simulink model "ugvmodel4point"  (R2025b)
settings: Solver=ode45  StartTime=0.0  StopTime=85  RelTol=1e-3
InitFcn:
  | UGVparameters
StopFcn:
  | myAnimation(xActEst,yActEst,thetaAct,X_array,Y_array,rp1,rp2)
  | myPlot(xActEst,yActEst,X_array,Y_array,rp1,rp2)
values from neighbouring files (symbols this model uses):
  b = 0.5842    [UGVparameters.m]
  rL = 0.052959    [UGVparameters.m]
  rR = 0.052959    [UGVparameters.m]
  wmax = Vmax/rR    (= 8.30831397874)    [UGVparameters.m]
settings Model: Creator=vigal  LastModifiedBy=brand
settings SolverCC: AlgebraicLoopSolver=TrustRegion
settings DataIOCC: ReturnWorkspaceOutputs=off
settings DebuggingCC: UnconnectedInputMsg=warning  UnconnectedOutputMsg=warning  UnconnectedLineMsg=warning  ArithmeticOperatorsInVariantConditions=warning
settings ModelReferenceCC: EnableRefExpFcnMdlSchedulingChecks=on
settings SFSimCC: SimUseLocalCustomCode=off  CustomCodeUndefinedFunction=UseInterfaceOnly
settings RTWCC: RTWUseLocalCustomCode=off  GPUComputeCapability=3.5

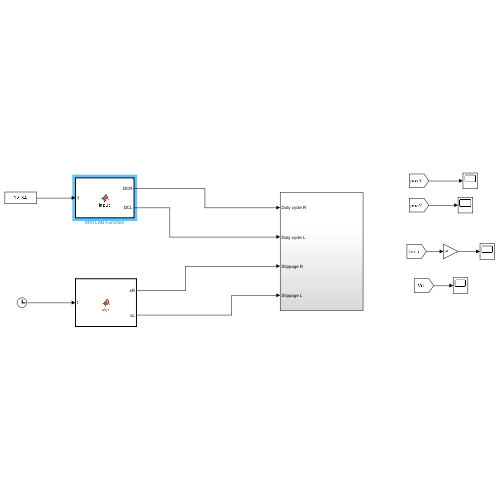
[thumbnail: Simulink's stored preview of the top-level diagram]
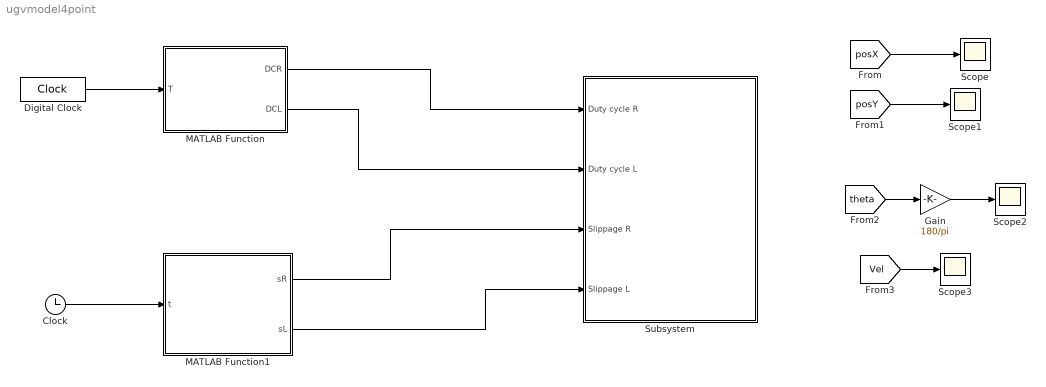
== system ugvmodel4point ==
  Clock : Clock
  Digital Clock : DigitalClock
  Gain : Gain  Gain=180/pi
  MATLAB Function : MATLAB Function  TreatAsAtomicUnit=on
  MATLAB Function1 : MATLAB Function  TreatAsAtomicUnit=on
  Scope{,1..3} (4 alike) : Scope
      Scope settings: ActiveDisplayYMinimum=-0.31428564567099693  ActiveDisplayYMaximum=2.8285708110389729  DataLoggingVariableName=xActEst
      Scope1 settings: ActiveDisplayYMinimum=-1.4039599693481954  ActiveDisplayYMaximum=1.2603387496671137  DataLoggingVariableName=yActEst
      Scope2 settings: ActiveDisplayYMinimum=-1.53363  ActiveDisplayYMaximum=13.80268  DataLoggingVariableName=thetaAct
      Scope3 settings: ActiveDisplayYMinimum=-0.055  ActiveDisplayYMaximum=0.49499  DataLoggingVariableName=ScopeData3
  Subsystem : Subsystem
  wires:
  Digital Clock/1 -> MATLAB Function/1(T)
  Clock/1 -> MATLAB Function1/1(t)
  MATLAB Function/1(DCR) -> Subsystem/1(Duty cycle R)
  MATLAB Function/2(DCL) -> Subsystem/2(Duty cycle L)
  MATLAB Function1/1(sR) -> Subsystem/3(Slippage R)
  MATLAB Function1/2(sL) -> Subsystem/4(Slippage L)
  [posX] -> Scope/1
  [theta] -> Gain/1
  [posY] -> Scope1/1
  [Vel] -> Scope3/1
  Gain/1 -> Scope2/1

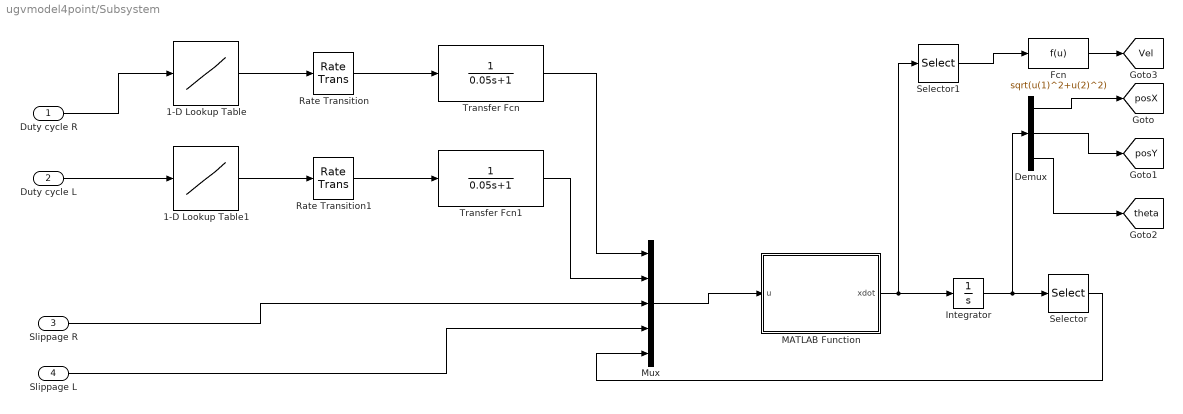
== system ugvmodel4point/Subsystem ==
  Duty cycle R : Inport
  Duty cycle L : Inport  Port=2
  Slippage R : Inport  Port=3
  Slippage L : Inport  Port=4
  1-D Lookup Table : Lookup_n-D  NumberOfTableDimensions=1  BreakpointsForDimension1=[-100 -30 0 30 100]  Table=[-wmax 0 0 0 wmax]  InternalRulePriority=Speed  RndMeth=Simplest
  1-D Lookup Table1 : Lookup_n-D  NumberOfTableDimensions=1  BreakpointsForDimension1=[-100 -30 0 30 100]  Table=[-wmax 0 0 0 wmax]  InternalRulePriority=Speed  RndMeth=Simplest
  Demux : Demux  Outputs=3
  Fcn : Fcn  Expr=sqrt(u(1)^2+u(2)^2)
  Integrator : Integrator  InitialCondition=[0;0;0]
  MATLAB Function : MATLAB Function  TreatAsAtomicUnit=on
  Mux : Mux  Inputs=5
  Rate Transition : RateTransition
  Rate Transition1 : RateTransition
  Selector : Selector  InputPortWidth=3  IndexOptions=Index vector (dialog)  Indices=[3]  OutputSizes=1
  Selector1 : Selector  InputPortWidth=3  IndexOptions=Index vector (dialog)  Indices=[1 2]  OutputSizes=1
  Transfer Fcn : TransferFcn  Denominator=[0.05 1]
  Transfer Fcn1 : TransferFcn  Denominator=[0.05 1]
  tag scope: Vel=global, posX=global, posY=global, theta=global
  wires:
  Slippage R/1 -> Mux/3
  1-D Lookup Table/1 -> Rate Transition/1
  Duty cycle R/1 -> 1-D Lookup Table/1
  Duty cycle L/1 -> 1-D Lookup Table1/1
  1-D Lookup Table1/1 -> Rate Transition1/1
  Rate Transition1/1 -> Transfer Fcn1/1
  Rate Transition/1 -> Transfer Fcn/1
  Transfer Fcn/1 -> Mux/1
  Slippage L/1 -> Mux/4
  Transfer Fcn1/1 -> Mux/2
  Mux/1 -> MATLAB Function/1(u)
  Integrator/1 -> Demux/1, Selector/1
  Selector/1 -> Mux/5
  Demux/1 -> [posX]
  Demux/3 -> [theta]
  Demux/2 -> [posY]
  MATLAB Function/1(xdot) -> Selector1/1, Integrator/1
  Selector1/1 -> Fcn/1
  Fcn/1 -> [Vel]

== matlab function ugvmodel4point/MATLAB Function1 ==
  data: t input; sR output; sL output
function [sR,sL] = slip(t)
%Simulation of the slippage factor on wheels

sR=0;
sL=0;

if t >= 15 && t < 18
    sR = 0.1;
    sL=0;

end

== matlab function ugvmodel4point/MATLAB Function ==
  data: T input; DCR output; DCL output
function [DCR,DCL] = input(T)
%Simulation of duty cycle percentage

%DCR -> duty cycle on right wheel
%DCL -> duty cycle on left wheel

DCR=0;
DCL=0;

if T >= 0 && T < 11
    DCR = 95;
    DCL = 95;

elseif T >= 15 && T < 18
    DCL = 100;  
    DCR = 51;

elseif T >= 25 && T < 35
    DCL = 93;   
    DCR = 93;
elseif T >= 40 && T < 43
    DCL = 99;   
    DCR = 50;
elseif T >= 50 && T < 60
    DCL = 95;  
    DCR = 95;
elseif T >= 65 && T < 68
    DCL = 100;  
    DCR = 52;
elseif T >= 70 && T < 81
    DCL = 95;  
    DCR = 95;
end

== matlab function ugvmodel4point/Subsystem/MATLAB Function ==
  data: u input; xdot output; rR parameter; rL parameter; b parameter
function xdot = ugv(u,rR, rL, b)

wR=u(1);
wL=u(2);
sR=u(3);
sL=u(4);
theta=u(5);

xdot=[((1-sL)*rL*wL+(1-sR)*rR*wR)*cos(theta)/2;...
       ((1-sL)*rL*wL+(1-sR)*rR*wR)*sin(theta)/2;...
       ((1-sL)*rL*wL-(1-sR)*rR*wR)/b];
